simulink model "bdot_static_test"  (R2016b)
settings: Solver=VariableStepAuto  StartTime=0.0  StopTime=10800  RelTol=1e-3  EnableMultiTasking=on
undefined symbols (not defined in the file or in its folder): sim_params
libraries: aerolibutil x2, dynamics_lib x2, bdot_controller_lib x1, command_processing x1, magnetometer_lib x1, magnetorquer_assembly_lib x1
settings Model: Creator=Taylor  LastModifiedBy=Taylor
settings OptimizationCC: DefaultParameterBehavior=Inlined  UseDivisionForNetSlopeComputation=on  UseFloatMulNetSlope=on  InlineInvariantSignals=on  PassReuseOutputArgsAs=Individual arguments  ZeroExternalMemoryAtStartup=off  ZeroInternalMemoryAtStartup=off  NoFixptDivByZeroProtection=on  EfficientFloat2IntCast=on  LifeSpan=1
settings DebuggingCC: ParameterTunabilityLossMsg=error  SFUnexpectedBacktrackingDiag=warning  SFNoUnconditionalDefaultTransitionDiag=warning  SFExecutionAtInitializationDiag=none
settings HardwareCC: ProdBitPerInt=16  ProdBitPerPointer=16  ProdBitPerSizeT=16  ProdBitPerPtrDiffT=16  ProdLargestAtomicFloat=None  ProdWordSize=16  ProdHWDeviceType=Texas Instruments->MSP430
settings RTWCC: SystemTargetFile=ert.tlc  TemplateMakefile=ert_default_tmf  Description=Embedded Coder  GenerateReport=on  IncludeHyperlinkInReport=on  LaunchReport=on  GenerateTraceInfo=on  GenerateTraceReport=on  GenerateTraceReportSl=on  GenerateTraceReportSf=on  GenerateTraceReportEml=on  GenerateCodeMetricsReport=on
settings CodeAppCC: ForceParamTrailComments=on  IgnoreCustomStorageClasses=off  OperatorAnnotations=on  SimulinkDataObjDesc=on  SFDataObjDesc=on  MATLABFcnDesc=on  CustomSymbolStrGlobalVar=rt$N$M  CustomSymbolStrType=$N$M  CustomSymbolStrFcn=$N$M$F  CustomSymbolStrMacro=$N$M  InsertBlockDesc=on  MATLABSourceComments=on
settings ERTTargetCC: GenerateSampleERTMain=on  CombineSignalStateStructs=on  SupportComplex=off  SupportContinuousTime=on  SupportNonInlinedSFcns=on  InlinedParameterPlacement=NonHierarchical  ERTCustomFileTemplate=example_file_process.tlc  ERTFilePackagingFormat=CompactWithDataFile
settings ConfigComp: CovMetricSettings=dw  CovHtmlReporting=on  CovSaveCumulativeToWorkspaceVar=on  CovSaveSingleToWorkspaceVar=on  CovExternalEMLEnable=off

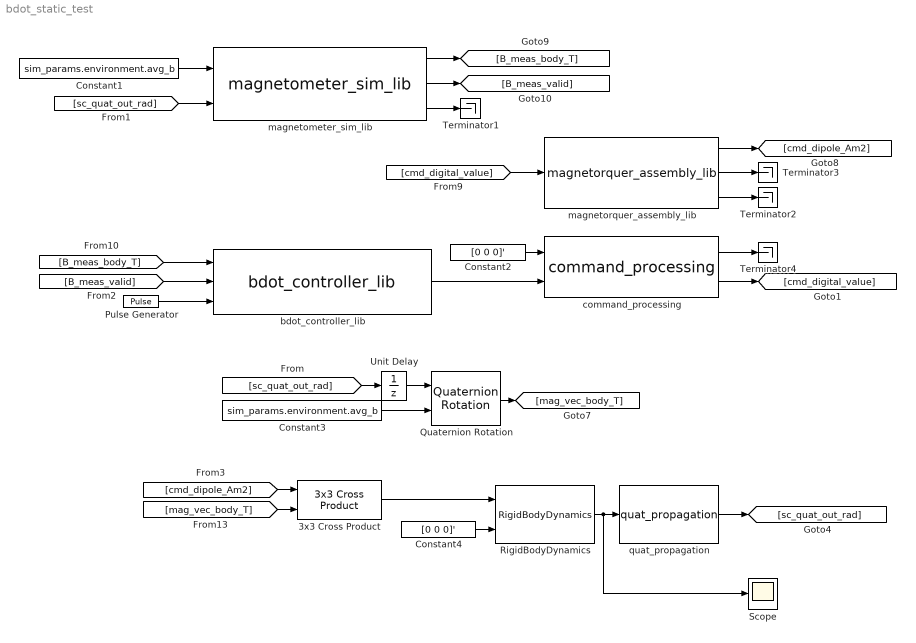
== system bdot_static_test ==
  3x3 Cross Product : aerolibutil/3x3 Cross Product
  Constant1 : Constant  Value=sim_params.environment.avg_b
  Constant2 : Constant  Value=[0 0 0]'
  Constant3 : Constant  Value=sim_params.environment.avg_b
  Constant4 : Constant  Value=[0 0 0]'
  Pulse Generator : DiscretePulseGenerator  PulseType=Time based  Period=sim_params.CAN.sync_pulse_s  PulseWidth=sim_params.actuators.pct_sync_pulse
  Quaternion Rotation : aerolibutil/Quaternion Rotation
  RigidBodyDynamics : dynamics_lib/Dynamics/RigidBodyDynamics
  Scope : Scope
  Terminator{1..4} (4 alike) : Terminator
  Unit Delay : UnitDelay  InitialCondition=[1;0;0;0]  SampleTime=-1
  bdot_controller_lib : bdot_controller_lib/bdot_controller_lib
  command_processing : command_processing/command_processing
  magnetometer_sim_lib : magnetometer_lib/magnetometer_sim_lib
  magnetorquer_assembly_lib : magnetorquer_assembly_lib/magnetorquer_assembly_lib
  quat_propagation : dynamics_lib/Dynamics/quat_propagation
  wires:
  [B_meas_body_T] -> bdot_controller_lib/1
  magnetometer_sim_lib/3 -> Terminator1/1
  magnetometer_sim_lib/1 -> [B_meas_body_T]
  magnetometer_sim_lib/2 -> [B_meas_valid]
  [sc_quat_out_rad] -> magnetometer_sim_lib/2
  Constant1/1 -> magnetometer_sim_lib/1
  [B_meas_valid] -> bdot_controller_lib/2
  Pulse Generator/1 -> bdot_controller_lib/3
  [cmd_digital_value] -> magnetorquer_assembly_lib/1
  magnetorquer_assembly_lib/1 -> [cmd_dipole_Am2]
  magnetorquer_assembly_lib/2 -> Terminator3/1
  magnetorquer_assembly_lib/3 -> Terminator2/1
  bdot_controller_lib/1 -> command_processing/2
  Constant2/1 -> command_processing/1
  command_processing/2 -> [cmd_digital_value]
  command_processing/1 -> Terminator4/1
  [mag_vec_body_T] -> 3x3 Cross Product/2
  [cmd_dipole_Am2] -> 3x3 Cross Product/1
  3x3 Cross Product/1 -> RigidBodyDynamics/1
  Constant4/1 -> RigidBodyDynamics/2
  RigidBodyDynamics/1 -> Scope/1, quat_propagation/1
  Unit Delay/1 -> Quaternion Rotation/1
  [sc_quat_out_rad] -> Unit Delay/1
  Quaternion Rotation/1 -> [mag_vec_body_T]
  Constant3/1 -> Quaternion Rotation/2
  quat_propagation/1 -> [sc_quat_out_rad]
